simulink model "ARM_project_final"  (R2018b)
settings: Solver=ode1  StartTime=0.0  StopTime=15  FixedStep=0.001  RelTol=1e-3
settings Model: Creator=2266716C  LastModifiedBy=sebis
settings DataIOCC: LimitDataPoints=on  SaveFormat=Array
settings OptimizationCC: BlockReduction=off  BooleanDataType=off  LifeSpan=inf
settings DebuggingCC: SaveWithParameterizedLinksMsg=none  UnderspecifiedInitializationDetection=Classic  MergeDetectMultiDrivingBlocksExec=none  SignalResolutionControl=TryResolveAllWithWarning  LibraryContextMissingDiagnostic=none  SFUnexpectedBacktrackingDiag=warning  SFNoUnconditionalDefaultTransitionDiag=warning  SFExecutionAtInitializationDiag=none
settings HardwareCC: ProdBitPerPointer=32  ProdBitPerSizeT=32  ProdBitPerPtrDiffT=32  ProdLargestAtomicFloat=None  ProdIntDivRoundTo=Undefined  ProdEndianess=Unspecified  ProdWordSize=32  ProdHWDeviceType=32-bit Generic  TargetUnknown=on
settings ModelReferenceCC: PropagateSignalLabelsOutOfModel=off
settings SFSimCC: SimUseLocalCustomCode=off
settings RTWCC: RTWUseLocalCustomCode=off
settings CodeAppCC: StateflowObjectComments=on
settings GRTTargetCC: TargetLangStandard=C89/C90 (ANSI)  GeneratePreprocessorConditionals=Disable all
settings ConfigComp: CovMetricSettings=dw  CovHtmlReporting=on  CovSaveCumulativeToWorkspaceVar=on  CovSaveSingleToWorkspaceVar=on  CovExternalEMLEnable=off  CovSFcnEnable=off

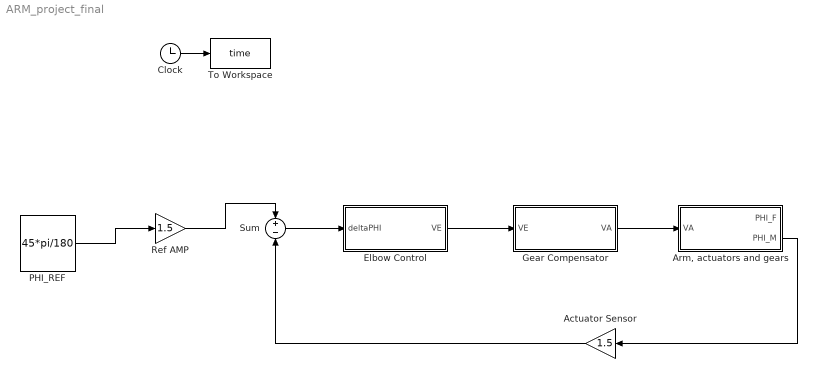
== system ARM_project_final ==
  Actuator Sensor : Gain  Gain=1.5
  "Arm, actuators and gears " : Subsystem
  Clock : Clock
  "Elbow Control " : Subsystem
  Gear Compensator : Subsystem
  PHI_REF : Constant  Value=45*pi/180
  "Ref AMP " : Gain  Gain=1.5
  Sum : Sum  Inputs=+-
  To Workspace : ToWorkspace  VariableName=time  SampleTime=-1
  wires:
  "Ref AMP "/1 -> Sum/1
  Actuator Sensor/1 -> Sum/2
  Sum/1 -> "Elbow Control "/1(deltaPHI)
  "Elbow Control "/1("VE ") -> Gear Compensator/1(VE)
  Gear Compensator/1(VA) -> "Arm, actuators and gears "/1("VA ")
  "Arm, actuators and gears "/2(PHI_M) -> Actuator Sensor/1
  PHI_REF/1 -> "Ref AMP "/1
  Clock/1 -> To Workspace/1

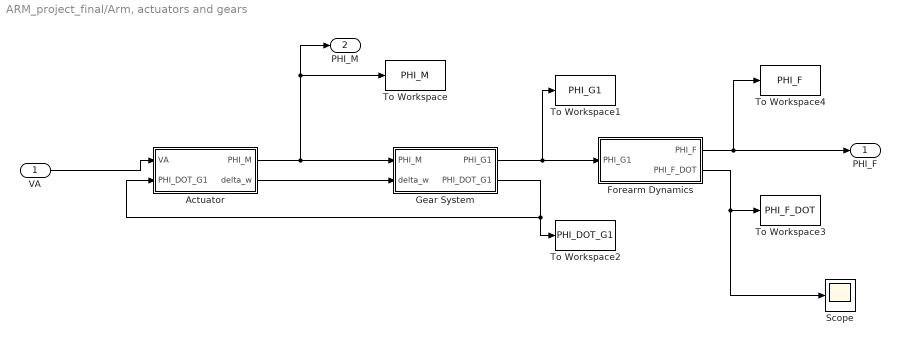
== system ARM_project_final/Arm, actuators and gears  ==
  "VA " : Inport
  Actuator : Subsystem
  "Forearm Dynamics " : Subsystem
  Gear System : Subsystem
  Scope : Scope
  To Workspace : ToWorkspace  VariableName=PHI_M  SampleTime=-1
  To Workspace1 : ToWorkspace  VariableName=PHI_G1  SampleTime=-1
  To Workspace2 : ToWorkspace  VariableName=PHI_DOT_G1  SampleTime=-1
      settings: Save2DSignal=2-D array (concatenate along first dimension)
  To Workspace3 : ToWorkspace  VariableName=PHI_F_DOT  SampleTime=-1
  To Workspace4 : ToWorkspace  VariableName=PHI_F  SampleTime=-1
  PHI_F : Outport
  PHI_M : Outport  Port=2
  wires:
  "VA "/1 -> Actuator/1("VA ")
  Actuator/2(delta_w) -> Gear System/2(delta_w)
  Gear System/1(PHI_G1) -> To Workspace1/1, "Forearm Dynamics "/1(PHI_G1)
  "Forearm Dynamics "/1("PHI_F ") -> To Workspace4/1, PHI_F/1
  Actuator/1("PHI_M ") -> To Workspace/1, PHI_M/1, Gear System/1(PHI_M)
  Gear System/2(PHI_DOT_G1) -> Actuator/2(PHI_DOT_G1), To Workspace2/1
  "Forearm Dynamics "/2("PHI_F_DOT ") -> Scope/1, To Workspace3/1

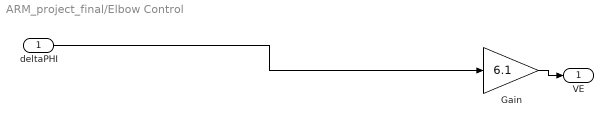
== system ARM_project_final/Elbow Control  ==
  deltaPHI : Inport
  Gain : Gain  Gain=6.1
  "VE " : Outport
  wires:
  Gain/1 -> "VE "/1
  deltaPHI/1 -> Gain/1

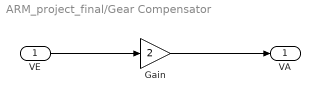
== system ARM_project_final/Gear Compensator ==
  VE : Inport
  Gain : Gain  Gain=2
  VA : Outport
  wires:
  VE/1 -> Gain/1
  Gain/1 -> VA/1

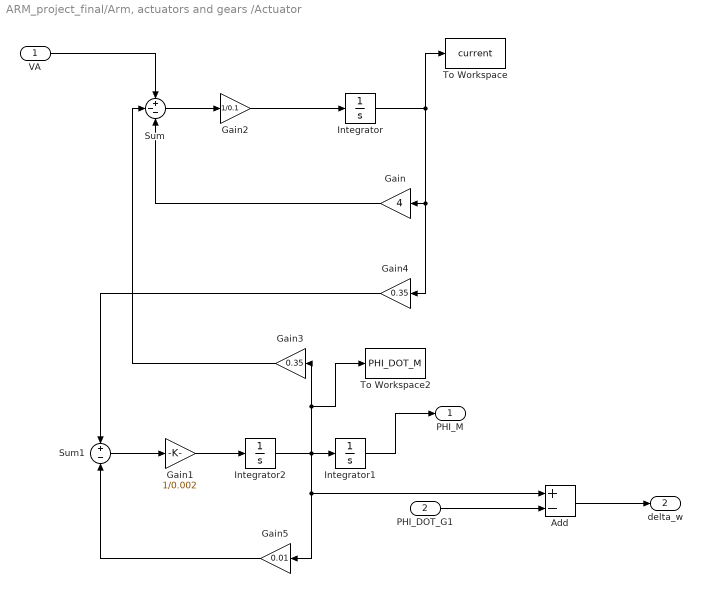
== system ARM_project_final/Arm, actuators and gears /Actuator ==
  "VA " : Inport
  PHI_DOT_G1 : Inport  Port=2
  Add : Sum  Inputs=+-
  Gain : Gain  Gain=4
  Gain1 : Gain  Gain=1/0.002
  Gain2 : Gain  Gain=1/0.1
  Gain3 : Gain  Gain=0.35
  Gain4 : Gain  Gain=0.35
  Gain5 : Gain  Gain=0.01
  Integrator : Integrator
  Integrator1 : Integrator
  Integrator2 : Integrator
  Sum : Sum  Inputs=+--
  Sum1 : Sum  Inputs=+-
  To Workspace : ToWorkspace  VariableName=current  SampleTime=-1
  To Workspace2 : ToWorkspace  VariableName=PHI_DOT_M  SampleTime=-1
      settings: Save2DSignal=2-D array (concatenate along first dimension)
  "PHI_M " : Outport
  delta_w : Outport  Port=2
  wires:
  Sum/1 -> Gain2/1
  Gain2/1 -> Integrator/1
  Integrator/1 -> Gain4/1, Gain/1, To Workspace/1
  Gain/1 -> Sum/3
  "VA "/1 -> Sum/1
  Integrator2/1 -> Add/1, Gain5/1, To Workspace2/1, Gain3/1, Integrator1/1
  Gain1/1 -> Integrator2/1
  Sum1/1 -> Gain1/1
  Gain5/1 -> Sum1/2
  Gain3/1 -> Sum/2
  Gain4/1 -> Sum1/1
  Integrator1/1 -> "PHI_M "/1
  Add/1 -> delta_w/1
  PHI_DOT_G1/1 -> Add/2

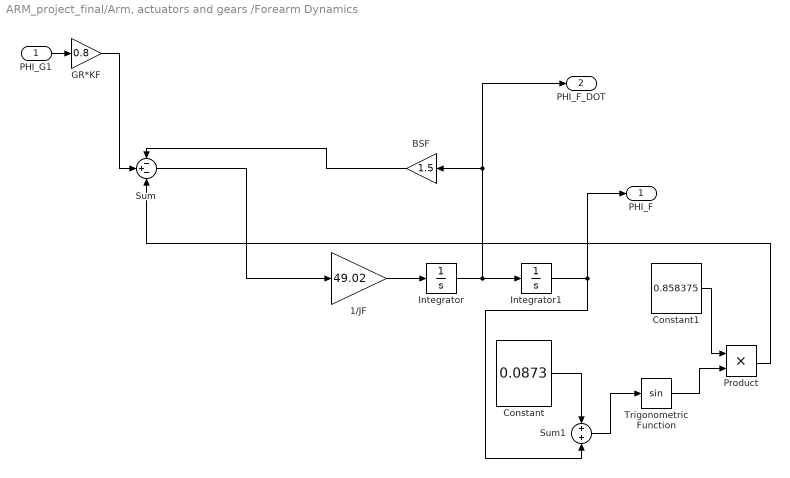
== system ARM_project_final/Arm, actuators and gears /Forearm Dynamics  ==
  PHI_G1 : Inport
  "1/JF " : Gain  Gain=49.02
  BSF : Gain  Gain=1.5
  Constant : Constant  Value=0.0873
  Constant1 : Constant  Value=0.858375
  GR*KF : Gain  Gain=0.8
  Integrator : Integrator
  Integrator1 : Integrator
  Product : Product
  Sum : Sum  Inputs=-+-
  Sum1 : Sum
  Trigonometric Function : Trigonometry  SampleTime=1
  "PHI_F " : Outport
  "PHI_F_DOT " : Outport  Port=2
  wires:
  PHI_G1/1 -> GR*KF/1
  GR*KF/1 -> Sum/2
  Integrator/1 -> "PHI_F_DOT "/1, BSF/1, Integrator1/1
  "1/JF "/1 -> Integrator/1
  Constant/1 -> Sum1/1
  Sum1/1 -> Trigonometric Function/1
  Integrator1/1 -> "PHI_F "/1, Sum1/2
  Trigonometric Function/1 -> Product/2
  Constant1/1 -> Product/1
  Product/1 -> Sum/3
  Sum/1 -> "1/JF "/1
  BSF/1 -> Sum/1

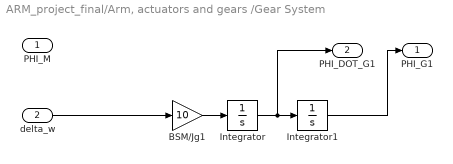
== system ARM_project_final/Arm, actuators and gears /Gear System ==
  PHI_M : Inport
  delta_w : Inport  Port=2
  BSM/Jg1 : Gain  Gain=10
  Integrator : Integrator
  Integrator1 : Integrator
  PHI_G1 : Outport
  PHI_DOT_G1 : Outport  Port=2
  wires:
  delta_w/1 -> BSM/Jg1/1
  BSM/Jg1/1 -> Integrator/1
  Integrator1/1 -> PHI_G1/1
  Integrator/1 -> PHI_DOT_G1/1, Integrator1/1
